simulink model "SimulinkProject"  (R2021a)
settings: Solver=VariableStepAuto  StartTime=0.0  StopTime=10.0  RelTol=1e-3
StartFcn:
  | learning.simulink.modelCallbacks.startFunction(gcs)
StopFcn:
  | learning.simulink.modelCallbacks.stopFunction(gcs)
model workspace (MAT data in the model file):
  courseObject.course = 'simulink'
  courseObject.chapter = 6
  courseObject.lesson = 1
  courseObject.section = 2
  courseObject.task = 1
  t_ans = [0; 0.1; 0.1; 0.2; 0.3; 0.4; 0.5; 0.6; 0.7; 0.8; 0.9; 1; 1.1; 1.1; 1.2; 1.2; 1.3; 1.4; 1.5; 1.6; 1.7; 1.8; 1.9; 2; 2; 2.1; 2.2; 2.3; 2.4; 2.5; 2.6; 2.7; 2.8; 2.9; 2.9; 3; 3.1; 3.2; 3.3; 3.4; 3.5; 3.6; 3.7; 3.8; 3.9; 4; 4.1; 4.2; 4.3; 4.4; 4.5; 4.6; 4.6; 4.7; 4.8; 4.9; 5; 5.1; 5.2; 5.2; 5.3; 5.4; 5.5; 5.6; 5.7; 5.8; 5.9; 6; 6; 6.1; 6.2; 6.3; 6.4; 6.5; 6.6; 6.7; 6.7; 6.8; 6.9; 7; 7.1; 7.2; 7.3; 7.4; 7.5; 7.6; 7.7; 7.7; 7.8; 7.9; 8; 8.1; 8.2; 8.3; 8.3; 8.4; 8.5; 8.6; 8.7; 8.8; 8.9; 9; 9.1; 9.2; 9.3; 9.4; 9.5; 9.6; 9.7; 9.8; 9.8; 9.9; 10]
  y_ans3 = [0; 0; 0; 0; 0; 0; 0; 0; 0; 0; 0; 0; 0; 0; 0; 1; 1; 1; 1; 1; 1; 1; 1; 1; 0; 0; 0; 0; 0; 0; 0; 0; 0; 0; 0; 0; 0; 0; 0; 0; 0; 0; 0; 0; 0; 0; 0; 0; 0; 0; 0; 0; 1; 1; 1; 1; 1; 1; 1; 0; 0; 0; 0; 0; 0; 0; 0; 0; 0; 0; 0; 0; 0; 0; 0; 0; 0; 0; 0; 0; 0; 0; 0; 0; 0; 0; 0; 0; 0; 0; 0; 0; 0; 0; 0; 0; 0; 0; 0; 0; 0; 0; 0; 0; 0; 0; 0; 0; 0; 0; 0; 0; 0]
  y_ans4 = [0; 0; 0; 0; 0; 0; 0; 0; 0; 0; 0; 0; 0; 0; 0; 1; 1; 1; 1; 1; 1; 1; 1; 1; 0; 0; 0; 0; 0; 0; 0; 0; 0; 0; 0; 0; 0; 0; 0; 0; 0; 0; 0; 0; 0; 0; 0; 0; 0; 0; 0; 0; 1; 1; 1; 1; 1; 1; 1; 0; 0; 0; 0; 0; 0; 0; 0; 0; 0; 0; 0; 0; 0; 0; 0; 0; 1; 1; 1; 1; 1; 1; 1; 1; 1; 1; 1; 0; 0; 0; 0; 0; 0; 0; 0; 0; 0; 0; 0; 0; 0; 0; 0; 0; 0; 0; 0; 0; 0; 0; 0; 0; 0]
  y_ans5 = [1; 1; 1; 1; 1; 1; 1; 1; 1; 1; 1; 1; 1; 1; 1; 2; 2; 2; 2; 2; 2; 2; 2; 2; 1; 1; 1; 1; 1; 1; 1; 1; 1; 1; 1; 1; 1; 1; 1; 1; 1; 1; 1; 1; 1; 1; 1; 1; 1; 1; 1; 1; 2; 2; 2; 2; 2; 2; 2; 1; 1; 1; 1; 1; 1; 1; 1; 1; 1; 1; 1; 1; 1; 1; 1; 1; 2; 2; 2; 2; 2; 2; 2; 2; 2; 2; 2; 1; 1; 1; 1; 1; 1; 1; 1; 1; 1; 1; 1; 1; 1; 1; 1; 1; 1; 1; 1; 1; 1; 1; 1; 1; 1]
libraries: simulink x3, SignalEditorBlockLib x1
CloseFcn:
  | learning.simulink.cleanupOnlineTraining
settings Model: Creator=HP  LastModifiedBy=HP
settings DataIOCC: SaveTime=off  OutputOption=SpecifiedOutputTimes  OutputTimes=t_ans

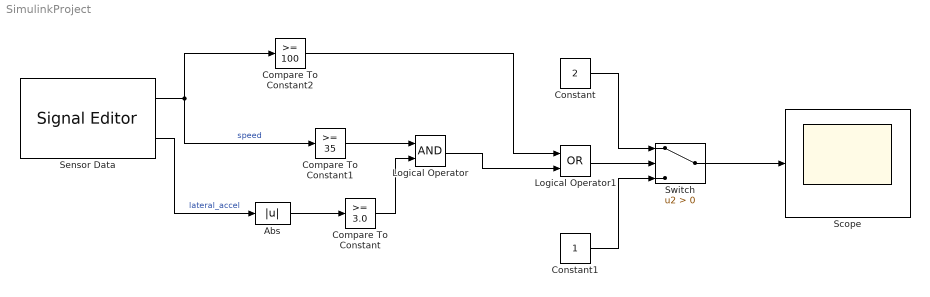
== system SimulinkProject ==
  Abs : Abs
  Compare To Constant : simulink/Logic and Bit Operations/Compare To Constant  relop=>=  const=3.0  OutDataTypeStr=boolean
  Compare To Constant1 : simulink/Logic and Bit Operations/Compare To Constant  relop=>=  const=35  OutDataTypeStr=boolean
  Compare To Constant2 : simulink/Logic and Bit Operations/Compare To Constant  relop=>=  const=100  OutDataTypeStr=boolean
  Constant : Constant  Value=2
  Constant1 : Constant
  Logical Operator : Logic  AllPortsSameDT=off  OutDataTypeStr=boolean
  Logical Operator1 : Logic  Operator=OR  AllPortsSameDT=off  OutDataTypeStr=boolean
  Scope : Scope
  Sensor Data : SignalEditorBlockLib/Signal Editor  FileName=signalData.mat  ActiveScenario=data  ActiveSignal=speed  IsBus=off  OutputBusObjectStr=Bus: BusObject  SampleTime=0  Interpolate=off  ZeroCross=off  OutputAfterFinalValue=Setting to zero  Unit=inherit  PreserveSignalName=on
  Switch : Switch  Criteria=u2 > Threshold
  wires:
  Sensor Data/1 -> Compare To Constant1/1, Compare To Constant2/1  "speed"
  Sensor Data/2 -> Abs/1  "lateral_accel"
  Abs/1 -> Compare To Constant/1
  Compare To Constant1/1 -> Logical Operator/1
  Compare To Constant/1 -> Logical Operator/2
  Compare To Constant2/1 -> Logical Operator1/1
  Logical Operator/1 -> Logical Operator1/2
  Switch/1 -> Scope/1
  Logical Operator1/1 -> Switch/2
  Constant1/1 -> Switch/3
  Constant/1 -> Switch/1
